simulink model "Tdof_robot_mdl"  (R2017b)
settings: Solver=FixedStepAuto  StartTime=0.0  StopTime=3  FixedStep=1e-4  RelTol=1e-4
libraries: simulink x4
settings Model: Creator=info  LastModifiedBy=info

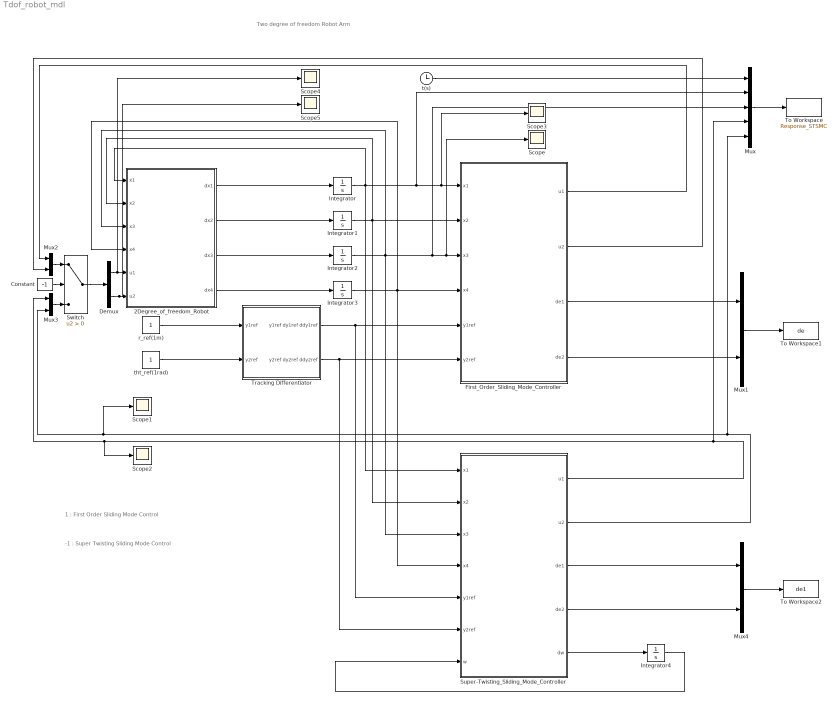
== system Tdof_robot_mdl ==
  note: Two degree of freedom Robot Arm
  note: 1 : First Order Sliding Mode Control
  note: -1 : Super Twisting Sliding Mode Control
  2Degree_of_freedom_Robot : MATLAB Function  TreatAsAtomicUnit=on
  Constant : Constant  Value=-1
  Demux : Demux  Outputs=2
  First_Order_Sliding_Mode_Controller : MATLAB Function  TreatAsAtomicUnit=on
  Integrator : Integrator  InitialCondition=0.001  AbsoluteTolerance=1e-4
  Integrator1 : Integrator  InitialCondition=0.001
  Integrator2 : Integrator
  Integrator3 : Integrator
  Integrator4 : Integrator
  Mux : Mux  Inputs=5
  Mux{1..4} (4 alike) : Mux  Inputs=2
  Scope{,1..5} (6 alike) : Scope
  Super-Twisting_Sliding_Mode_Controller : MATLAB Function  TreatAsAtomicUnit=on
  Switch : Switch  Criteria=u2 > Threshold
  To Workspace : ToWorkspace  VariableName=Response_STSMC  SaveFormat=Timeseries  SampleTime=-1
      settings: Save2DSignal=2-D array (concatenate along first dimension)
  To Workspace1 : ToWorkspace  VariableName=de  SaveFormat=Timeseries  SampleTime=-1
      settings: Save2DSignal=2-D array (concatenate along first dimension)
  To Workspace2 : ToWorkspace  VariableName=de1  SaveFormat=Timeseries  SampleTime=-1
      settings: Save2DSignal=2-D array (concatenate along first dimension)
  Tracking Differentiator : Subsystem
  r_ref(1m) : Constant
  t(s) : Clock
  tht_ref(1rad) : Constant
  wires:
  2Degree_of_freedom_Robot/2(dx2) -> Integrator1/1
  2Degree_of_freedom_Robot/3(dx3) -> Integrator2/1
  2Degree_of_freedom_Robot/4(dx4) -> Integrator3/1
  2Degree_of_freedom_Robot/1(dx1) -> Integrator/1
  Integrator3/1 -> Super-Twisting_Sliding_Mode_Controller/4(x4), 2Degree_of_freedom_Robot/4(x4), First_Order_Sliding_Mode_Controller/4(x4)
  First_Order_Sliding_Mode_Controller/4(de2) -> Mux1/2
  First_Order_Sliding_Mode_Controller/1(u1) -> Mux2/1
  First_Order_Sliding_Mode_Controller/2(u2) -> Mux2/2
  r_ref(1m)/1 -> Tracking Differentiator/1(y1ref)
  tht_ref(1rad)/1 -> Tracking Differentiator/2(y2ref)
  Tracking Differentiator/2(y2ref dy2ref ddy2ref) -> Super-Twisting_Sliding_Mode_Controller/6(y2ref), First_Order_Sliding_Mode_Controller/6(y2ref)
  Tracking Differentiator/1(y1ref dy1ref ddy1ref) -> Super-Twisting_Sliding_Mode_Controller/5(y1ref), First_Order_Sliding_Mode_Controller/5(y1ref)
  Integrator2/1 -> Super-Twisting_Sliding_Mode_Controller/3(x3), 2Degree_of_freedom_Robot/3(x3), Scope/1, First_Order_Sliding_Mode_Controller/3(x3), Mux/3
  Mux/1 -> To Workspace/1
  t(s)/1 -> Mux/1
  Mux1/1 -> To Workspace1/1
  First_Order_Sliding_Mode_Controller/3(de1) -> Mux1/1
  Mux2/1 -> Switch/1
  Demux/2 -> Scope5/1, 2Degree_of_freedom_Robot/6(u2)
  Demux/1 -> Scope4/1, 2Degree_of_freedom_Robot/5(u1)
  Switch/1 -> Demux/1
  Mux3/1 -> Switch/3
  Mux4/1 -> To Workspace2/1
  Super-Twisting_Sliding_Mode_Controller/1(u1) -> Mux/4, Scope2/1, Mux3/1
  Constant/1 -> Switch/2
  Integrator/1 -> 2Degree_of_freedom_Robot/1(x1), Scope3/1, First_Order_Sliding_Mode_Controller/1(x1), Mux/2, Super-Twisting_Sliding_Mode_Controller/1(x1)
  Integrator1/1 -> Super-Twisting_Sliding_Mode_Controller/2(x2), 2Degree_of_freedom_Robot/2(x2), First_Order_Sliding_Mode_Controller/2(x2)
  Integrator4/1 -> Super-Twisting_Sliding_Mode_Controller/7(w)
  Super-Twisting_Sliding_Mode_Controller/2(u2) -> Mux/5, Scope1/1, Mux3/2
  Super-Twisting_Sliding_Mode_Controller/3(de1) -> Mux4/1
  Super-Twisting_Sliding_Mode_Controller/4(de2) -> Mux4/2
  Super-Twisting_Sliding_Mode_Controller/5(dw) -> Integrator4/1

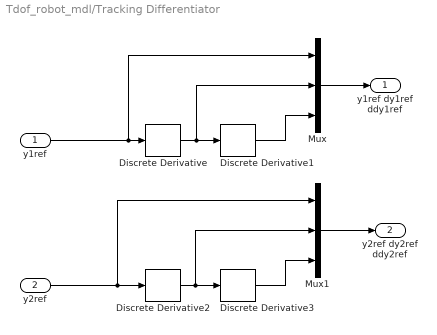
== system Tdof_robot_mdl/Tracking Differentiator ==
  y1ref : Inport
  y2ref : Inport  Port=2
  Discrete Derivative{,1..3} (4 alike) : simulink/Discrete/Discrete Derivative  gainval=eps  ICPrevScaledInput=0.0  OutMin=[]  OutMax=[]  OutDataType=fixdt(1, 16)  OutScaling=2^-10  DoSatur=off
  Mux : Mux  Inputs=3
  Mux1 : Mux  Inputs=3
  y1ref dy1ref ddy1ref : Outport
  y2ref dy2ref ddy2ref : Outport  Port=2
  wires:
  Discrete Derivative/1 -> Mux/2, Discrete Derivative1/1
  y1ref/1 -> Mux/1, Discrete Derivative/1
  Discrete Derivative2/1 -> Mux1/2, Discrete Derivative3/1
  y2ref/1 -> Mux1/1, Discrete Derivative2/1
  Discrete Derivative1/1 -> Mux/3
  Mux/1 -> y1ref dy1ref ddy1ref/1
  Discrete Derivative3/1 -> Mux1/3
  Mux1/1 -> y2ref dy2ref ddy2ref/1

== matlab function Tdof_robot_mdl/First_Order_Sliding_Mode_Controller ==
  data: x1 input; u1 output; x2 input; x3 input; x4 input; y1ref input size=3; y2ref input size=3; u2 output; de1 output; de2 output
function [u1,u2,de1,de2] = FOSMC(x1,x2,x3,x4,y1ref,y2ref)
%% Manipulator Mass and Gravity
m = 1; g = 9.8;
%% Attractivity and Stability constants for sliding surface
k1 = 10; k2 = 10;
lambda1 = 5; lambda2 = 5;
y1 = x1;
y2 = x3;
dy1 = x2;
dy2 = x4;
dy1ref = y1ref(2);
dy2ref = y2ref(2);
ddy1ref = y1ref(3);
ddy2ref = y2ref(3);
%% Errors and their derivatives
e1 = y1-y1ref(1);
e2 = y2-y2ref(1);
de1 = dy1-dy1ref;
de2 = dy2-dy2ref;
%% Sliding surfaces
s1 = de1+lambda1*e1;
s2 = de2+lambda2*e2;
%% Control law : u = ueq+udisc
u1 = m*(-x1*x4^2+g*sin(x3)+ddy1ref-lambda1*de1-k1*sign(s1));
u2 = m*x1^2*(1/x1*(2*x2*x4+g*cos(x3))-lambda2*de2+ddy2ref-k2*sign(s2));
end

== matlab function Tdof_robot_mdl/2Degree_of_freedom_Robot ==
  data: x1 input; dx1 output; x2 input; x3 input; x4 input; u1 input; u2 input; dx2 output; dx3 output; dx4 output
function [dx1,dx2,dx3,dx4]= Tdof_robot(x1,x2,x3,x4,u1,u2)
m = 1; g = 9.8;
dx1 = x2;
dx2 = x1*x4^2-g*sin(x3)+u1/m;
dx3 = x4;
dx4 = 1/x1^2*(-2*x1*x2*x4-g*x1*cos(x3)+u2/m);
end

== matlab function Tdof_robot_mdl/Super-Twisting_Sliding_Mode_Controller ==
  data: x1 input; u1 output; x2 input; x3 input; x4 input; y1ref input size=3; y2ref input size=3; w input size=2; u2 output; de1 output; de2 output; dw output size=2
function [u1,u2,de1,de2,dw] = STSMC(x1,x2,x3,x4,y1ref,y2ref,w)
%% Manipulator Mass and Gravity
m = 1; g = 9.8;
%% Attractivity and Stability constants for sliding surface
lambda1 = 3; lambda2 = 3;
y1 = x1;
y2 = x3;
dy1 = x2;
dy2 = x4;
dy1ref = y1ref(2);
dy2ref = y2ref(2);
ddy1ref = y1ref(3);
ddy2ref = y2ref(3);
%% Errors and their derivatives
e1 = y1-y1ref(1);
e2 = y2-y2ref(1);
de1 = dy1-dy1ref;
de2 = dy2-dy2ref;
%% Sliding surfaces
s1 = de1+lambda1*e1;
s2 = de2+lambda2*e2;
%% Super-Twisting Algorithm
F = 50;     % Tuning Parameter
T = 50;     % Tuning Parameter
dw = [-1.1*F*sign(s1);-1.1*T*sign(s2)];
u1dis = -sqrt(F)*sqrt(abs(s1))*sign(s1)+w(1);
u2dis = -sqrt(T)*sqrt(abs(s2))*sign(s2)+w(2);
u1 = m*(-x1*x4^2+g*sin(x3)+ddy1ref-lambda1*de1+u1dis);
u2 = m*x1^2*(1/x1*(2*x2*x4+g*cos(x3))-lambda2*de2+ddy2ref+u2dis);
end
